simulink model "simulink_full_system"  (R2025b)
settings: Solver=VariableStepAuto  StartTime=0.0  StopTime=10  FixedStep=0.001  RelTol=1e-3
values from neighbouring files (symbols this model uses):
  Ts = 0.01    [PID_konstants.m]    (also in simulink_PI.m)
settings Model: Creator=fred441a  LastModifiedBy=fred441a
settings SolverCC: ConcurrentTasks=on

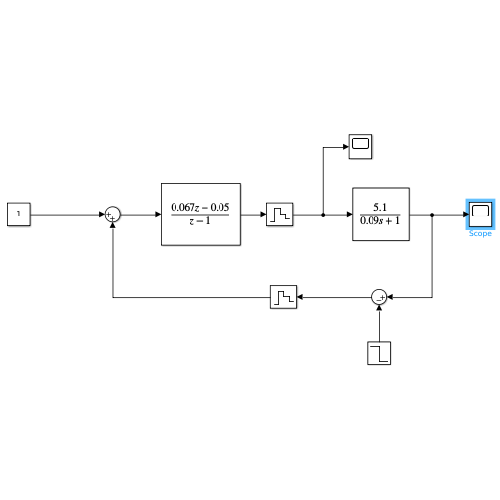
[thumbnail: Simulink's stored preview of the top-level diagram]
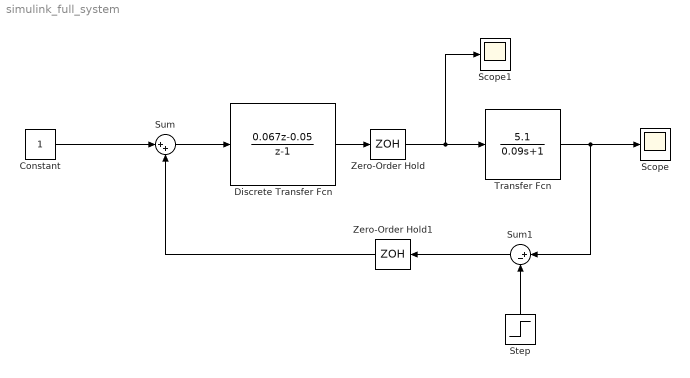
== system simulink_full_system ==
  Constant : Constant
  Discrete Transfer Fcn : DiscreteTransferFcn  Numerator=[0.067,-0.05]  Denominator=[1 ,-1]
  Scope : Scope
      settings: ActiveDisplayYMinimum=-9.8628532149441863  ActiveDisplayYMaximum=8.9272603245328153
  Scope1 : Scope
      settings: ActiveDisplayYMinimum=-0.042734094447703819  ActiveDisplayYMaximum=2.1544465388946579
  Step : Step  Time=5  After=-0.02  SampleTime=0
  Sum : Sum  Inputs=|++
  Sum1 : Sum  Inputs=|+-
  Transfer Fcn : TransferFcn  Numerator=[5.1]  Denominator=[0.09,1]
  Zero-Order Hold : ZeroOrderHold  SampleTime=Ts
  Zero-Order Hold1 : ZeroOrderHold  SampleTime=Ts
  wires:
  Zero-Order Hold/1 -> Scope1/1, Transfer Fcn/1
  Transfer Fcn/1 -> Sum1/1, Scope/1
  Discrete Transfer Fcn/1 -> Zero-Order Hold/1
  Constant/1 -> Sum/1
  Sum/1 -> Discrete Transfer Fcn/1
  Zero-Order Hold1/1 -> Sum/2
  Sum1/1 -> Zero-Order Hold1/1
  Step/1 -> Sum1/2
